simulink model "Hardware_Diagnostics_Test"  (R2025b)
settings: Solver=FixedStepDiscrete  StartTime=0.0  StopTime=inf  FixedStep=50e-6  RelTol=1e-3  EnableMultiTasking=on
undefined symbols (not defined in the file or in its folder): bit, Down, GPTRIP1SEL, GPTRIP2SEL, TZ1, TZ2, Up
libraries: c2802xlib x5, c280xlib x3, c2806xlib x2

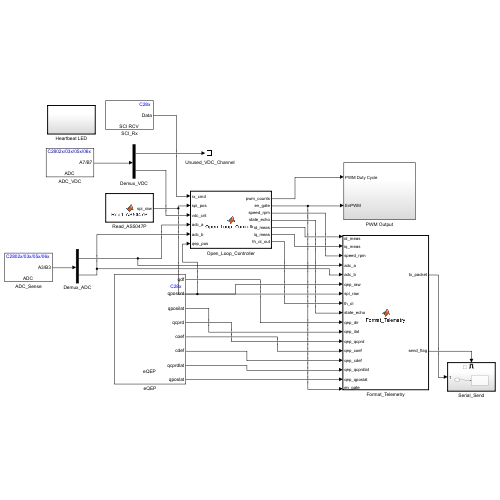
[thumbnail: Simulink's stored preview of the top-level diagram]
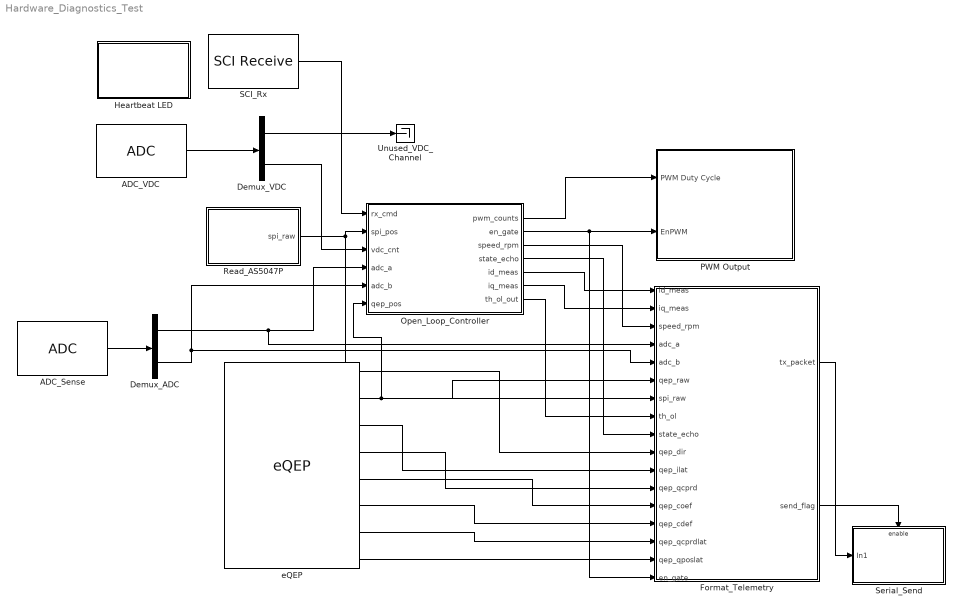
== system Hardware_Diagnostics_Test ==
  ADC_Sense : c2802xlib/ADC  blkParamProc=C2000  ADCModule=1  samplingMode=Simultaneous sample mode  ADCResolution=12-bit (Single-ended input)  ADC29xResolution=12-bit  ADCMode=Single-ended input  useSOC1=SOC0  useSOC2=SOC0_SOC1  SOCAcquisitionWindow=7  SOCTriggerSource=ePWM4_ADCSOCA  SOCInterruptTrigger=No ADCINT  Ts=-1  dType=uint16  postInterrupt=on  interruptSel=ADCINT1  ADCINTContinuous=on  endma=off  chdma=1  conv1=ADCINA0  conv2=ADCINA3 and ADCINB3  conv1_Type4=ADCIN0  conv2_Type4=ADCIN0 and ADCIN1
  ADC_VDC : c2802xlib/ADC  blkParamProc=C2000  ADCModule=1  samplingMode=Simultaneous sample mode  ADCResolution=12-bit (Single-ended input)  ADC29xResolution=12-bit  ADCMode=Single-ended input  useSOC1=SOC2  useSOC2=SOC2_SOC3  SOCAcquisitionWindow=7  SOCTriggerSource=Software  SOCInterruptTrigger=No ADCINT  Ts=-1  dType=uint16  postInterrupt=off  interruptSel=ADCINT1  ADCINTContinuous=on  endma=off  chdma=1  conv1=ADCINB7  conv2=ADCINA7 and ADCINB7  conv1_Type4=ADCIN0  conv2_Type4=ADCIN0 and ADCIN1
  Demux_ADC : Demux  Outputs=2
  Demux_VDC : Demux  Outputs=2
  Format_Telemetry : MATLAB Function  TreatAsAtomicUnit=on
  Heartbeat LED : Subsystem  TreatAsAtomicUnit=on
  Open_Loop_Controller : MATLAB Function  TreatAsAtomicUnit=on
  PWM Output : Subsystem
  Read_AS5047P : MATLAB Function  TreatAsAtomicUnit=on
  SCI_Rx : c280xlib/SCI Receive  Priority=2  sciModule=A  dataHead=''  headerCheckMaxCount=16  dataTail=''  dataType=uint8  dataLenOptions=Length via dialog  dataDim=1  maxDataLength=1  initValue=0  errOption=Output the last received value  errValue=0  sampleTime=-1  blockingMode=off  timeOut=inf  outputStatus=off
  Serial_Send : Subsystem
  Unused_VDC_Channel : Terminator
  eQEP : c280xlib/eQEP  useModule=eQEP1  pcInputmode=Quadrature-count  externalClockrate=2x resolution: Count the rising/falling edge  swapPolarityselection=Counterclockwise  qdfOutputport=on  qapPolarityselection=off  qbpPolarityselection=off  qipPolarityselection=off  qspPolarityselection=off  igatePolarityselection=off  sampleTime=-1  pcOutputport=on  pcMaximumvalue=4095  indexInitializationcheck=off  indexInitializationevent=Falling edge  strobeInitializationcheck=off  strobeInitializationevent=Rising edge  softwareInitializationcheck=off  softwareInitializationsource=Set to init value at start up  softwareInitializationmode=on  pcInitialvalue=0  pcResetmode=Reset on the maximum position  ieloutputport=on  indexEventlatch=Rising edge  seloutputport=off  strobeEventlatch=Rising edge  pcefOutputport=on  enableEqepcapture=on  qctmrOutputport=off  qcprdOutputport=on  captureTimerprescaler=128  upEventprescaler=128  overflowErrorflag=on  directionErrorflag=on  captureTimerposition=On position counter read  unitTimerperiod=100000000  captureTimerlatch=off  capturePeriodlatch=on  positionCounterlatch=on  soenPolarityselection=off  spselPolarityselection=Index pin is used for sync output  compareValuesource=Specify via dialog  shadowMode=Load on QPOSCNT=0  compareValue=4294967295  syncOutputwidth=1  polaritySyncoutput=Active high  watchdogEnable=on  watchdogTimer=65535  outport1Datatype=auto  outport2Datatype=auto  outport3Datatype=auto  outport4Datatype=auto  outport5Datatype=auto  outport6Datatype=auto  outport7Datatype=auto  outport8Datatype=auto  outport9Datatype=auto  outport10Datatype=auto  outport11Datatype=auto  outport12Datatype=auto  eqepinterrupt_pce=on  eqepinterrupt_qpe=on  eqepinterrupt_qdc=on  eqepinterrupt_wto=on  eqepinterrupt_pcu=off  eqepinterrupt_pco=off  eqepinterrupt_pcr=off  eqepinterrupt_pcm=off  eqepinterrupt_sel=off  eqepinterrupt_iel=on  eqepinterrupt_uto=on  pheOutputport=on  watchdogOutputport=on  outport13Datatype=auto  outport14Datatype=auto
  wires:
  ADC_VDC/1 -> Demux_VDC/1
  Demux_VDC/2 -> Open_Loop_Controller/3(vdc_cnt)
  SCI_Rx/1 -> Open_Loop_Controller/1(rx_cmd)
  Open_Loop_Controller/5(id_meas) -> Format_Telemetry/1(id_meas)
  Demux_VDC/1 -> Unused_VDC_Channel/1
  Read_AS5047P/1(spi_raw) -> Format_Telemetry/7(spi_raw), Open_Loop_Controller/2(spi_pos)
  Open_Loop_Controller/1(pwm_counts) -> PWM Output/1(PWM Duty Cycle)
  Open_Loop_Controller/2(en_gate) -> Format_Telemetry/17(en_gate), PWM Output/2(EnPWM)
  Open_Loop_Controller/7(th_ol_out) -> Format_Telemetry/8(th_ol)
  Open_Loop_Controller/3(speed_rpm) -> Format_Telemetry/3(speed_rpm)
  Open_Loop_Controller/4(state_echo) -> Format_Telemetry/9(state_echo)
  Open_Loop_Controller/6(iq_meas) -> Format_Telemetry/2(iq_meas)
  Format_Telemetry/1(tx_packet) -> Serial_Send/1(In1)
  Format_Telemetry/2(send_flag) -> Serial_Send/Enable
  eQEP/8 -> Format_Telemetry/16(qep_qposlat)
  eQEP/6 -> Format_Telemetry/14(qep_cdef)
  eQEP/3 -> Format_Telemetry/11(qep_ilat)
  eQEP/1 -> Format_Telemetry/10(qep_dir)
  eQEP/2 -> Format_Telemetry/6(qep_raw), Open_Loop_Controller/6(qep_pos)
  eQEP/4 -> Format_Telemetry/12(qep_qcprd)
  eQEP/7 -> Format_Telemetry/15(qep_qcprdlat)
  Demux_ADC/1 -> Format_Telemetry/4(adc_a), Open_Loop_Controller/4(adc_a)
  Demux_ADC/2 -> Format_Telemetry/5(adc_b), Open_Loop_Controller/5(adc_b)
  eQEP/5 -> Format_Telemetry/13(qep_coef)
  ADC_Sense/1 -> Demux_ADC/1

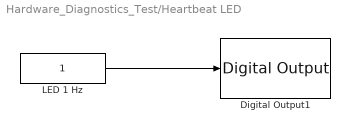
== system Hardware_Diagnostics_Test/Heartbeat LED ==
  Digital Output1 : c2806xlib/Digital Output  GPIO_Number=GPIO32~GPIO39  GPIO_Bit0=off  GPIO_BIT0_Toggle=off  GPIO_Bit1=off  GPIO_BIT1_Toggle=off  GPIO_Bit2=on  GPIO_BIT2_Toggle=on  GPIO_Bit3=off  GPIO_BIT3_Toggle=off  GPIO_Bit4=off  GPIO_BIT4_Toggle=off  GPIO_Bit5=off  GPIO_BIT5_Toggle=off  GPIO_Bit6=off  GPIO_BIT6_Toggle=off  GPIO_Bit7=off  GPIO_BIT7_Toggle=off
  LED 1 Hz : Constant  OutDataTypeStr=uint16  SampleTime=0.5
  wires:
  LED 1 Hz/1 -> Digital Output1/1

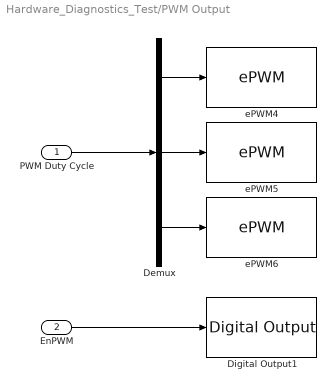
== system Hardware_Diagnostics_Test/PWM Output ==
  PWM Duty Cycle : Inport
  EnPWM : Inport  Port=2
  Demux : Demux  Outputs=3
  Digital Output1 : c2806xlib/Digital Output  GPIO_Number=GPIO50~GPIO55  GPIO_Bit0=off  GPIO_BIT0_Toggle=off  GPIO_Bit1=off  GPIO_BIT1_Toggle=off  GPIO_Bit2=on  GPIO_BIT2_Toggle=off  GPIO_Bit3=off  GPIO_BIT3_Toggle=off  GPIO_Bit4=off  GPIO_BIT4_Toggle=off  GPIO_Bit5=off  GPIO_BIT5_Toggle=off  GPIO_Bit6=off  GPIO_BIT6_Toggle=off  GPIO_Bit7=off  GPIO_BIT7_Toggle=off
  ePWM4 : c2802xlib/ePWM  PwmType=C2000  useModule=ePWM4  ePWMxLINKTBPRD=Not Linked  periodUnits=Clock cycles  timerSource=Specify via dialog  timerPeriod_clk=2250  timerPeriod_sec=64000  tbshadow=Counter equals to zero  countingMode=Up-Down  phaseActiveEnable=Disable  phaseDirection=Count down after sync  phaseActive=0  synchronizationEnable=off  dcaevt1Sync=off  dcbevt1Sync=off  synchronizationOption=Counter equals to zero (CTR=Zero)  dcbevt1SyncOut=off  dcaevt1SyncOut=off  cmpdSyncOut=off  cmpcSyncOut=off  cmpbSyncOut=off  zeroSyncOut=on  swfSyncOut=off  perSynchronizationOption=Counter equals to period (CTR=PRD)  clockPrescale=1  HSclockPrescale=1  enswap=off  ePWMxAStatus=on  ePWMxAactionLogic1=Do nothing  ePWMxAactionLogic2=Do nothing  ePWMxAactionLogic3=Clear  ePWMxAactionLogic4=Set  ePWMxAactionLogic5=Do nothing  ePWMxAactionLogic6=Do nothing  ePWMxACSFenable=off  ePWMxACSFvalue=Forcing disable  ePWMxASFreload=Zero  ePWMxBStatus=off  ePWMxBactionLogic1=Do nothing  ePWMxBactionLogic2=Set  ePWMxBactionLogic3=Do nothing  ePWMxBactionLogic4=Do nothing  ePWMxBactionLogic5=Clear  ePWMxBactionLogic6=Do nothing  ePWMxBCSFenable=off  ePWMxBCSFvalue=Forcing disable  ePWMxBSFreload=Zero  ePWNxBOutWay=off  ePWMxLINKCMPA=Not Linked  CMPAUnits=Clock cycles  CMPASource=Input port  CMPAValue_per=32000  CMPAValue_clk=1125  enCMPAshadow=Counter equals to zero (CTR=Zero)  ePWMxLINKCMPB=Not Linked  CMPBUnits=Clock cycles  CMPBSource=Specify via dialog  CMPBValue_per=50  CMPBValue_clk=1125  enCMPBshadow=Counter equals to zero (CTR=Zero)  ePWMxLINKCMPC=Not Linked  CMPCUnits=Clock cycles  CMPCSource=Specify via dialog  CMPCValue_per=50  CMPCValue_clk=32000  enCMPCshadow=Counter equals to zero (CTR=Zero)  ePWMxLINKCMPD=Not Linked  CMPDUnits=Clock cycles  CMPDSource=Specify via dialog  CMPDValue_per=50  CMPDValue_clk=32000  enCMPDshadow=Counter equals to zero (CTR=Zero)  enableDBePWMxA=on  enableDBePWMxB=on  enhalfcycle=off  DBpolarity=Active high complementary (AHC)  DBedgeDelay=Positive  DBSource_ePWMxA=ePWMxA  DBSource_ePWMxB=ePWMxA  DBPeriodUnits=Clock cycles  DBperiodSource=Specify via dialog  REDperiod=5  FEDperiod=5  REDperiod_sec=0  FEDperiod_sec=0  LoadModeDBRED=Immediate without using shadow  LoadModeDBFED=Immediate without using shadow  adcstartModuleA=on  adcrequestEventA=First event  adcstartEventA=Counter equals to period (CTR=PRD)  adcstartEventA_type2=Digital Compare Module A Event 1 start of conversion (DCAEVT1.soc)  adcstartModuleB=off  adcrequestEventB=First event  adcstartEventB=Counter equals to zero (CTR=Zero)  adcstartEventB_type2=Counter equals to zero (CTR=Zero)  intEn=off  intPrd=First event  intSel=Counter equals to zero (CTR=Zero)  intSel_type2=Counter equals to zero (CTR=Zero)  hrpe=off  enHRPWM=off  HRPWM_LoadMode=Counter equals to period (CTR=PRD)  HRPWM_CTLMode=Duty or Period control mode  HRPWM_EDGMode=Both edge  hrpeb=off  enHRPWMB=off  HRPWM_LoadModeB=Counter equals to zero (CTR=ZERO)  HRPWM_CTLModeB=Duty or Period control mode  HRPWM_EDGModeB=Both edge  enHRDBRED=off  enHRDBFED=off  enSFO=on  enautoconv=on  chopperEnable=off  chopperFrequency=1  chopperFirstwidth=1  chopperDuty=12.5%  tripZonesource=Specify via dialog  tzselOSHT1=off  tzselOSHT2=off  tzselOSHT3=off  tzselOSHT4=off  tzselOSHT5=off  tzselOSHT6=off  tzselOSHDCAEV1=off  tzselOSHDCBEV1=off  tzselCBC1=off  tzselCBC2=off  tzselCBC3=off  tzselCBC4=off  tzselCBC5=off  tzselCBC6=off  tzselCBCDCAEV2=off  tzselCBCDCBEV2=off  enTzOstIntr=off  enTzCbcIntr=off  enTzDCAEVT1Intr=off  enTzDCAEVT2Intr=off  enTzDCBEVT1Intr=off  enTzDCBEVT2Intr=off  tzclrCBCLatch=Counter equals to zero (CTR=Zero)  ePWMxAforced=No action  ePWMxBforced=No action  DCAEVT1forced=No action  DCBEVT1forced=No action  DCAEVT2forced=No action  DCBEVT2forced=No action  dcah=Trip Zone 1 input (TZ1)  dcal=Trip Zone 2 input (TZ2)  dcbh=Trip Zone 1 input (TZ1)  dcbl=Trip Zone 2 input (TZ2)  dcah_type2=GPTRIP1SEL/(TZ1)  dcal_type2=GPTRIP2SEL/(TZ2)  dcbh_type2=GPTRIP1SEL/(TZ1)  dcbl_type2=GPTRIP2SEL/(TZ2)  gendcaevt1=Event disabled  gendcaevt2=Event disabled  gendcbevt1=Event disabled  gendcbevt2=Event disabled  dcaevt1src=DCAEVT1 with sync  dcaevt2src=DCAEVT2 with sync  dcbevt1src=DCBEVT1 with sync  dcbevt2src=DCBEVT2 with sync  pulsesel=Counter equals to zero (CTR=Zero)  blankinv=off  blankoffset=0  blankwidth=0  evsrcsel=Filtered version of DCAEVT1 (DCAEVT1FILT)  encape=off
  ePWM5 : c2802xlib/ePWM  PwmType=C2000  useModule=ePWM5  ePWMxLINKTBPRD=Not Linked  periodUnits=Clock cycles  timerSource=Specify via dialog  timerPeriod_clk=2250  timerPeriod_sec=64000  tbshadow=Counter equals to zero  countingMode=Up-Down  phaseActiveEnable=Set counter to phase value specified via dialog  phaseDirection=Count up after sync  phaseActive=0  synchronizationEnable=off  dcaevt1Sync=off  dcbevt1Sync=off  synchronizationOption=Pass through (EPWMxSYNCI or SWFSYNC)  dcbevt1SyncOut=off  dcaevt1SyncOut=off  cmpdSyncOut=off  cmpcSyncOut=off  cmpbSyncOut=off  zeroSyncOut=off  swfSyncOut=on  perSynchronizationOption=Counter equals to period (CTR=PRD)  clockPrescale=1  HSclockPrescale=1  enswap=off  ePWMxAStatus=on  ePWMxAactionLogic1=Do nothing  ePWMxAactionLogic2=Do nothing  ePWMxAactionLogic3=Clear  ePWMxAactionLogic4=Set  ePWMxAactionLogic5=Do nothing  ePWMxAactionLogic6=Do nothing  ePWMxACSFenable=off  ePWMxACSFvalue=Forcing disable  ePWMxASFreload=Zero  ePWMxBStatus=off  ePWMxBactionLogic1=Do nothing  ePWMxBactionLogic2=Set  ePWMxBactionLogic3=Do nothing  ePWMxBactionLogic4=Do nothing  ePWMxBactionLogic5=Clear  ePWMxBactionLogic6=Do nothing  ePWMxBCSFenable=off  ePWMxBCSFvalue=Forcing disable  ePWMxBSFreload=Zero  ePWNxBOutWay=off  ePWMxLINKCMPA=Not Linked  CMPAUnits=Clock cycles  CMPASource=Input port  CMPAValue_per=32000  CMPAValue_clk=1125  enCMPAshadow=Counter equals to zero (CTR=Zero)  ePWMxLINKCMPB=Not Linked  CMPBUnits=Clock cycles  CMPBSource=Specify via dialog  CMPBValue_per=50  CMPBValue_clk=1125  enCMPBshadow=Counter equals to zero (CTR=Zero)  ePWMxLINKCMPC=Not Linked  CMPCUnits=Clock cycles  CMPCSource=Specify via dialog  CMPCValue_per=50  CMPCValue_clk=32000  enCMPCshadow=Counter equals to zero (CTR=Zero)  ePWMxLINKCMPD=Not Linked  CMPDUnits=Clock cycles  CMPDSource=Specify via dialog  CMPDValue_per=50  CMPDValue_clk=32000  enCMPDshadow=Counter equals to zero (CTR=Zero)  enableDBePWMxA=on  enableDBePWMxB=on  enhalfcycle=off  DBpolarity=Active high complementary (AHC)  DBedgeDelay=Positive  DBSource_ePWMxA=ePWMxA  DBSource_ePWMxB=ePWMxA  DBPeriodUnits=Clock cycles  DBperiodSource=Specify via dialog  REDperiod=5  FEDperiod=5  REDperiod_sec=0  FEDperiod_sec=0  LoadModeDBRED=Immediate without using shadow  LoadModeDBFED=Immediate without using shadow  adcstartModuleA=off  adcrequestEventA=First event  adcstartEventA=Digital Compare Module A Event 1 start of conversion (DCAEVT1.soc)  adcstartEventA_type2=Digital Compare Module A Event 1 start of conversion (DCAEVT1.soc)  adcstartModuleB=off  adcrequestEventB=First event  adcstartEventB=Counter equals to zero (CTR=Zero)  adcstartEventB_type2=Counter equals to zero (CTR=Zero)  intEn=off  intPrd=First event  intSel=Counter equals to zero (CTR=Zero)  intSel_type2=Counter equals to zero (CTR=Zero)  hrpe=off  enHRPWM=off  HRPWM_LoadMode=Counter equals to period (CTR=PRD)  HRPWM_CTLMode=Duty or Period control mode  HRPWM_EDGMode=Both edge  hrpeb=off  enHRPWMB=off  HRPWM_LoadModeB=Counter equals to zero (CTR=ZERO)  HRPWM_CTLModeB=Duty or Period control mode  HRPWM_EDGModeB=Both edge  enHRDBRED=off  enHRDBFED=off  enSFO=on  enautoconv=on  chopperEnable=off  chopperFrequency=1  chopperFirstwidth=1  chopperDuty=12.5%  tripZonesource=Specify via dialog  tzselOSHT1=off  tzselOSHT2=off  tzselOSHT3=off  tzselOSHT4=off  tzselOSHT5=off  tzselOSHT6=off  tzselOSHDCAEV1=off  tzselOSHDCBEV1=off  tzselCBC1=off  tzselCBC2=off  tzselCBC3=off  tzselCBC4=off  tzselCBC5=off  tzselCBC6=off  tzselCBCDCAEV2=off  tzselCBCDCBEV2=off  enTzOstIntr=off  enTzCbcIntr=off  enTzDCAEVT1Intr=off  enTzDCAEVT2Intr=off  enTzDCBEVT1Intr=off  enTzDCBEVT2Intr=off  tzclrCBCLatch=Counter equals to zero (CTR=Zero)  ePWMxAforced=No action  ePWMxBforced=No action  DCAEVT1forced=No action  DCBEVT1forced=No action  DCAEVT2forced=No action  DCBEVT2forced=No action  dcah=Trip Zone 1 input (TZ1)  dcal=Trip Zone 2 input (TZ2)  dcbh=Trip Zone 1 input (TZ1)  dcbl=Trip Zone 2 input (TZ2)  dcah_type2=GPTRIP1SEL/(TZ1)  dcal_type2=GPTRIP2SEL/(TZ2)  dcbh_type2=GPTRIP1SEL/(TZ1)  dcbl_type2=GPTRIP2SEL/(TZ2)  gendcaevt1=Event disabled  gendcaevt2=Event disabled  gendcbevt1=Event disabled  gendcbevt2=Event disabled  dcaevt1src=DCAEVT1 with sync  dcaevt2src=DCAEVT2 with sync  dcbevt1src=DCBEVT1 with sync  dcbevt2src=DCBEVT2 with sync  pulsesel=Counter equals to zero (CTR=Zero)  blankinv=off  blankoffset=0  blankwidth=0  evsrcsel=Filtered version of DCAEVT1 (DCAEVT1FILT)  encape=off
  ePWM6 : c2802xlib/ePWM  PwmType=C2000  useModule=ePWM6  ePWMxLINKTBPRD=Not Linked  periodUnits=Clock cycles  timerSource=Specify via dialog  timerPeriod_clk=2250  timerPeriod_sec=64000  tbshadow=Counter equals to zero  countingMode=Up-Down  phaseActiveEnable=Set counter to phase value specified via dialog  phaseDirection=Count up after sync  phaseActive=0  synchronizationEnable=off  dcaevt1Sync=off  dcbevt1Sync=off  synchronizationOption=Disable  dcbevt1SyncOut=off  dcaevt1SyncOut=off  cmpdSyncOut=off  cmpcSyncOut=off  cmpbSyncOut=off  zeroSyncOut=off  swfSyncOut=off  perSynchronizationOption=Counter equals to period (CTR=PRD)  clockPrescale=1  HSclockPrescale=1  enswap=off  ePWMxAStatus=on  ePWMxAactionLogic1=Do nothing  ePWMxAactionLogic2=Do nothing  ePWMxAactionLogic3=Clear  ePWMxAactionLogic4=Set  ePWMxAactionLogic5=Do nothing  ePWMxAactionLogic6=Do nothing  ePWMxACSFenable=off  ePWMxACSFvalue=Forcing disable  ePWMxASFreload=Zero  ePWMxBStatus=off  ePWMxBactionLogic1=Do nothing  ePWMxBactionLogic2=Set  ePWMxBactionLogic3=Do nothing  ePWMxBactionLogic4=Do nothing  ePWMxBactionLogic5=Clear  ePWMxBactionLogic6=Do nothing  ePWMxBCSFenable=off  ePWMxBCSFvalue=Forcing disable  ePWMxBSFreload=Zero  ePWNxBOutWay=off  ePWMxLINKCMPA=Not Linked  CMPAUnits=Clock cycles  CMPASource=Input port  CMPAValue_per=32000  CMPAValue_clk=1125  enCMPAshadow=Counter equals to zero (CTR=Zero)  ePWMxLINKCMPB=Not Linked  CMPBUnits=Clock cycles  CMPBSource=Specify via dialog  CMPBValue_per=50  CMPBValue_clk=1125  enCMPBshadow=Counter equals to zero (CTR=Zero)  ePWMxLINKCMPC=Not Linked  CMPCUnits=Clock cycles  CMPCSource=Specify via dialog  CMPCValue_per=50  CMPCValue_clk=32000  enCMPCshadow=Counter equals to zero (CTR=Zero)  ePWMxLINKCMPD=Not Linked  CMPDUnits=Clock cycles  CMPDSource=Specify via dialog  CMPDValue_per=50  CMPDValue_clk=32000  enCMPDshadow=Counter equals to zero (CTR=Zero)  enableDBePWMxA=on  enableDBePWMxB=on  enhalfcycle=off  DBpolarity=Active high complementary (AHC)  DBedgeDelay=Positive  DBSource_ePWMxA=ePWMxA  DBSource_ePWMxB=ePWMxA  DBPeriodUnits=Clock cycles  DBperiodSource=Specify via dialog  REDperiod=5  FEDperiod=5  REDperiod_sec=0  FEDperiod_sec=0  LoadModeDBRED=Immediate without using shadow  LoadModeDBFED=Immediate without using shadow  adcstartModuleA=off  adcrequestEventA=First event  adcstartEventA=Digital Compare Module A Event 1 start of conversion (DCAEVT1.soc)  adcstartEventA_type2=Digital Compare Module A Event 1 start of conversion (DCAEVT1.soc)  adcstartModuleB=off  adcrequestEventB=First event  adcstartEventB=Counter equals to zero (CTR=Zero)  adcstartEventB_type2=Counter equals to zero (CTR=Zero)  intEn=off  intPrd=First event  intSel=Counter equals to zero (CTR=Zero)  intSel_type2=Counter equals to zero (CTR=Zero)  hrpe=off  enHRPWM=off  HRPWM_LoadMode=Counter equals to period (CTR=PRD)  HRPWM_CTLMode=Duty or Period control mode  HRPWM_EDGMode=Both edge  hrpeb=off  enHRPWMB=off  HRPWM_LoadModeB=Counter equals to zero (CTR=ZERO)  HRPWM_CTLModeB=Duty or Period control mode  HRPWM_EDGModeB=Both edge  enHRDBRED=off  enHRDBFED=off  enSFO=on  enautoconv=on  chopperEnable=off  chopperFrequency=1  chopperFirstwidth=1  chopperDuty=12.5%  tripZonesource=Specify via dialog  tzselOSHT1=off  tzselOSHT2=off  tzselOSHT3=off  tzselOSHT4=off  tzselOSHT5=off  tzselOSHT6=off  tzselOSHDCAEV1=off  tzselOSHDCBEV1=off  tzselCBC1=off  tzselCBC2=off  tzselCBC3=off  tzselCBC4=off  tzselCBC5=off  tzselCBC6=off  tzselCBCDCAEV2=off  tzselCBCDCBEV2=off  enTzOstIntr=off  enTzCbcIntr=off  enTzDCAEVT1Intr=off  enTzDCAEVT2Intr=off  enTzDCBEVT1Intr=off  enTzDCBEVT2Intr=off  tzclrCBCLatch=Counter equals to zero (CTR=Zero)  ePWMxAforced=No action  ePWMxBforced=No action  DCAEVT1forced=No action  DCBEVT1forced=No action  DCAEVT2forced=No action  DCBEVT2forced=No action  dcah=Trip Zone 1 input (TZ1)  dcal=Trip Zone 2 input (TZ2)  dcbh=Trip Zone 1 input (TZ1)  dcbl=Trip Zone 2 input (TZ2)  dcah_type2=GPTRIP1SEL/(TZ1)  dcal_type2=GPTRIP2SEL/(TZ2)  dcbh_type2=GPTRIP1SEL/(TZ1)  dcbl_type2=GPTRIP2SEL/(TZ2)  gendcaevt1=Event disabled  gendcaevt2=Event disabled  gendcbevt1=Event disabled  gendcbevt2=Event disabled  dcaevt1src=DCAEVT1 with sync  dcaevt2src=DCAEVT2 with sync  dcbevt1src=DCBEVT1 with sync  dcbevt2src=DCBEVT2 with sync  pulsesel=Counter equals to zero (CTR=Zero)  blankinv=off  blankoffset=0  blankwidth=0  evsrcsel=Filtered version of DCAEVT1 (DCAEVT1FILT)  encape=off
  wires:
  Demux/1 -> ePWM4/1
  Demux/2 -> ePWM5/1
  PWM Duty Cycle/1 -> Demux/1
  Demux/3 -> ePWM6/1
  EnPWM/1 -> Digital Output1/1

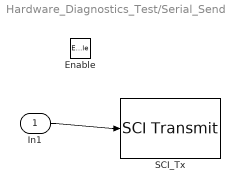
== system Hardware_Diagnostics_Test/Serial_Send ==
  In1 : Inport
  Enable : EnablePort
  SCI_Tx : c280xlib/SCI Transmit  sciModule=A  dataHead='S'  dataTail='E'  frameSize=1  blockingMode=on  outputStatus=off
  wires:
  In1/1 -> SCI_Tx/1

== matlab function Hardware_Diagnostics_Test/Read_AS5047P ==
function spi_raw = Read_AS5047P()
%#codegen
% SPI-A AS5047P read on GPIO16/17/18 with GPIO19 chip select.
% Force the EPC91200 PWM trip before the first controller update.
persistent init_done
spi_raw = uint16(0);
if coder.target('Rtw')
    coder.cinclude('as5047p_spi.h');
    coder.cinclude('pwm_gate_control.h');
    coder.updateBuildInfo('addSourceFiles', 'as5047p_spi.c');
    coder.updateBuildInfo('addSourceFiles', 'pwm_gate_control.c');
    coder.updateBuildInfo('addIncludePaths', 'C:\\96v_gan_humanoid_drive\\phase1\\simulation\\MyFOC code');
    if isempty(init_done)
        coder.ceval('pwm_gate_control', uint16(0));
        coder.ceval('as5047p_spi_init');
        init_done = true;
    end
    coder.ceval('as5047p_spi_read', coder.ref(spi_raw));
end
end

== matlab function Hardware_Diagnostics_Test/Format_Telemetry ==
function [tx_packet, send_flag] = Format_Telemetry(id_meas, iq_meas, speed_rpm, adc_a, adc_b, qep_raw, spi_raw, th_ol, state_echo, qep_dir, qep_ilat, qep_qcprd, qep_coef, qep_cdef, qep_qcprdlat, qep_qposlat, en_gate)
%#codegen
persistent dec_cnt
if isempty(dec_cnt), dec_cnt=uint16(0); end
dec_cnt=dec_cnt+uint16(1);
if dec_cnt>=uint16(20), dec_cnt=uint16(0); send_flag=true; else, send_flag=false; end

tx_packet=zeros(33,1,'uint8');
id_u16=typecast(int16(round(id_meas*single(100.0))),'uint16');
iq_u16=typecast(int16(round(iq_meas*single(100.0))),'uint16');
spd_u16=typecast(int16(round(speed_rpm)),'uint16');
aa=uint16(adc_a); ab=uint16(adc_b); spi_val=uint16(spi_raw); qep_val=uint16(qep_raw); ilat_val=uint16(qep_ilat);
th_norm=th_ol*single(10430.37835); if th_norm<single(0.0), th_norm=single(0.0); end; if th_norm>single(65535.0), th_norm=single(65535.0); end; th_u16=uint16(th_norm);
qcprd_val=uint16(qep_qcprd); coef_val=uint16(qep_coef); cdef_val=uint16(qep_cdef); qcprdlat_val=uint16(qep_qcprdlat); qposlat_val=uint16(qep_qposlat);

tx_packet(1)=uint8(83); tx_packet(2)=uint8(170); tx_packet(3)=uint8(85);
tx_packet(4)=uint8(bitshift(id_u16,-8)); tx_packet(5)=uint8(bitand(id_u16,255)); tx_packet(6)=uint8(bitshift(iq_u16,-8)); tx_packet(7)=uint8(bitand(iq_u16,255)); tx_packet(8)=uint8(bitshift(spd_u16,-8)); tx_packet(9)=uint8(bitand(spd_u16,255));
tx_packet(10)=uint8(bitshift(aa,-8)); tx_packet(11)=uint8(bitand(aa,255)); tx_packet(12)=uint8(bitshift(ab,-8)); tx_packet(13)=uint8(bitand(ab,255)); tx_packet(14)=uint8(bitshift(spi_val,-8)); tx_packet(15)=uint8(bitand(spi_val,255)); tx_packet(16)=uint8(bitshift(qep_val,-8)); tx_packet(17)=uint8(bitand(qep_val,255));
tx_packet(18)=uint8(bitshift(ilat_val,-8)); tx_packet(19)=uint8(bitand(ilat_val,255)); tx_packet(20)=uint8(qep_dir~=0); tx_packet(21)=uint8(qep_coef~=0); tx_packet(22)=uint8(qep_cdef~=0);
tx_packet(23)=uint8(bitshift(qcprd_val,-8)); tx_packet(24)=uint8(bitand(qcprd_val,255)); tx_packet(25)=uint8(bitshift(qcprdlat_val,-8)); tx_packet(26)=uint8(bitand(qcprdlat_val,255)); tx_packet(27)=uint8(bitshift(qposlat_val,-8)); tx_packet(28)=uint8(bitand(qposlat_val,255));
tx_packet(29)=uint8(bitshift(th_u16,-8)); tx_packet(30)=uint8(bitand(th_u16,255)); tx_packet(31)=uint8(state_echo); tx_packet(32)=uint8(en_gate); tx_packet(33)=uint8(69);
end

== matlab function Hardware_Diagnostics_Test/Open_Loop_Controller ==
function [pwm_counts, en_gate, speed_rpm, state_echo, id_meas, iq_meas, th_ol_out] = Open_Loop_Controller(rx_cmd, spi_pos, vdc_cnt, adc_a, adc_b, qep_pos)
%#codegen
% BOARD-SIDE COMMISSIONING CONTROLLER
%
% Commands:
%   0/S/s : stop and latch the ePWM software trip
%   A/a/4 : apply a small static alignment vector and capture both encoders
%   P/p/5 : open-loop electrical rotation in the board-positive direction
%   N/n/7 : open-loop electrical rotation in the board-negative direction
%   C/c   : clear the captured QEP electrical offset and stop
%
% SPI is sampled during alignment as an independent absolute reference.
% QEP is the runtime mechanical angle/speed source after calibration.
% The dashboard does not alter any of these signs.

pwm_counts = single([1125.0;1125.0;1125.0]);
en_gate = false;
speed_rpm = single(0.0);
state_echo = uint8(0);
id_meas = single(0.0);
iq_meas = single(0.0);
th_ol_out = single(0.0);

persistent state align_timer sample_count sum_spi_sin sum_spi_cos ...
    sum_qep_sin sum_qep_cos qep_elec_offset cal_valid spd_timer ...
    last_qep filt_speed qep_speed_initialized theta_ol last_cmd

if isempty(state)
    state = uint8(0);
    align_timer = uint32(0);
    sample_count = uint32(0);
    sum_spi_sin = single(0.0);
    sum_spi_cos = single(0.0);
    sum_qep_sin = single(0.0);
    sum_qep_cos = single(0.0);
    qep_elec_offset = single(0.0);
    cal_valid = false;
    spd_timer = uint16(0);
    last_qep = uint16(0);
    filt_speed = single(0.0);
    qep_speed_initialized = false;
    theta_ol = single(0.0);
    last_cmd = uint8(0);
end

TWO_PI = single(6.283185307);
TWO_PI_OVER_3 = single(2.094395102);
POLE_PAIRS = single(21.0);
SPI_COUNTS_PER_REV = single(16384.0);
QEP_COUNTS_PER_REV = int32(4096);
QEP_HALF_REV = int32(2048);
QEP_ANGLE_SCALE = TWO_PI / single(4096.0);
QEP_RPM_SCALE = single(14.6484375);       % 4096 counts/rev, 1 ms update
TS_FAST = single(0.00005);                 % 20 kHz controller step
PWM_PERIOD = single(2250.0);

ALIGN_HOLD_TICKS = uint32(30000);          % 1.5 s
ALIGN_SETTLE_TICKS = uint32(20000);        % collect after first 1.0 s
ALIGN_MIN_SAMPLES = uint32(500);
ALIGN_MODULATION = single(0.01);            % intentionally conservative
OPEN_LOOP_MODULATION = single(0.02);        % first powered test only
OPEN_LOOP_MECH_RPM = single(2.0);            % deliberately slow bench test
OPEN_LOOP_ELEC_SPEED = OPEN_LOOP_MECH_RPM * POLE_PAIRS * TWO_PI / single(60.0);
ALIGN_CURRENT_LIMIT = single(1.0);          % board ADC units must be verified
MIN_VDC = single(30.0);

% Convert board ADC channels to the existing diagnostic current estimate.
vdc_volts = single(vdc_cnt) * single(3.3 * 46.4545 / 4095.0);
offset_a = single(2041.0);
offset_b = single(2059.0);
I_SCALE = single(-0.02014652);
ia = (single(adc_a) - offset_a) * I_SCALE;
ib = (single(adc_b) - offset_b) * I_SCALE;
i_alpha = ia;
i_beta = (ia + single(2.0) * ib) * single(0.577350269);
i_mag = sqrt(i_alpha * i_alpha + i_beta * i_beta);

% Raw encoder angles. QEP polarity was configured in the model so the
% hand-spin-positive direction is the board-positive direction.
spi_i32 = mod(int32(spi_pos), int32(16384));
if spi_i32 < int32(0), spi_i32 = spi_i32 + int32(16384); end
theta_spi = single(spi_i32) / SPI_COUNTS_PER_REV * TWO_PI;

qep_i32 = mod(int32(qep_pos), QEP_COUNTS_PER_REV);
if qep_i32 < int32(0), qep_i32 = qep_i32 + QEP_COUNTS_PER_REV; end
theta_qep = single(qep_i32) * QEP_ANGLE_SCALE;

% QEP speed with a first-sample guard so startup cannot create false RPM.
if ~qep_speed_initialized
    last_qep = uint16(qep_i32);
    qep_speed_initialized = true;
end
spd_timer = spd_timer + uint16(1);
if spd_timer >= uint16(20)
    spd_timer = uint16(0);
    delta_qep = qep_i32 - int32(last_qep);
    if delta_qep > QEP_HALF_REV
        delta_qep = delta_qep - QEP_COUNTS_PER_REV;
    elseif delta_qep < -QEP_HALF_REV
        delta_qep = delta_qep + QEP_COUNTS_PER_REV;
    end
    last_qep = uint16(qep_i32);
    filt_speed = single(0.85) * filt_speed + ...
        single(0.15) * single(delta_qep) * QEP_RPM_SCALE;
end
speed_rpm = filt_speed;

% Process command bytes. A zero/no-byte result is ignored so a command
% remains latched until the next explicit command or STOP.
last_state = state;
% Execute each recognized serial command once. This prevents a held SCI byte
% from restarting alignment on every 50 us step.
if rx_cmd ~= last_cmd
    if rx_cmd == uint8(48) || rx_cmd == uint8(83) || rx_cmd == uint8(115)
        state = uint8(0);
        last_cmd = rx_cmd;
    elseif rx_cmd == uint8(65) || rx_cmd == uint8(97) || rx_cmd == uint8(52)
        state = uint8(4);
        last_cmd = rx_cmd;
    elseif rx_cmd == uint8(80) || rx_cmd == uint8(112) || rx_cmd == uint8(53)
        state = uint8(5);
        last_cmd = rx_cmd;
    elseif rx_cmd == uint8(78) || rx_cmd == uint8(110) || rx_cmd == uint8(55)
        state = uint8(7);
        last_cmd = rx_cmd;
    elseif rx_cmd == uint8(67) || rx_cmd == uint8(99)
        state = uint8(0);
        cal_valid = false;
        qep_elec_offset = single(0.0);
        theta_ol = single(0.0);
        last_cmd = rx_cmd;
    end
end

if state ~= last_state
    if state == uint8(4)
        align_timer = uint32(0);
        sample_count = uint32(0);
        sum_spi_sin = single(0.0);
        sum_spi_cos = single(0.0);
        sum_qep_sin = single(0.0);
        sum_qep_cos = single(0.0);
    elseif state == uint8(5) || state == uint8(7)
        % Start at the measured QEP electrical position so a re-run after
        % a hand movement is deterministic.
        theta_qep_e = mod(POLE_PAIRS * theta_qep + qep_elec_offset + TWO_PI, TWO_PI);
        theta_ol = theta_qep_e;
    end
end

% Runtime electrical angle from calibrated QEP. This is intentionally not
% derived from SPI during the open-loop test.
theta_qep_e = mod(POLE_PAIRS * theta_qep + qep_elec_offset + TWO_PI, TWO_PI);
cos_qep_e = cos(theta_qep_e);
sin_qep_e = sin(theta_qep_e);
id_meas = i_alpha * cos_qep_e + i_beta * sin_qep_e;
iq_meas = -i_alpha * sin_qep_e + i_beta * cos_qep_e;

if state == uint8(4)
    state_echo = uint8(4);
    if vdc_volts < MIN_VDC
        state_echo = uint8(13);             % requested alignment, no HV bus
        en_gate = false;
        pwm_counts = single([1125.0;1125.0;1125.0]);
    elseif i_mag > ALIGN_CURRENT_LIMIT
        state = uint8(11);
        state_echo = uint8(11);
        en_gate = false;
        pwm_counts = single([1125.0;1125.0;1125.0]);
    else
        align_timer = align_timer + uint32(1);

        % Static positive phase-A vector: electrical zero for this test.
        da = single(0.5) + ALIGN_MODULATION;
        db = single(0.5) - ALIGN_MODULATION * single(0.5);
        dc = db;
        pwm_counts = [da * PWM_PERIOD; db * PWM_PERIOD; dc * PWM_PERIOD];
        en_gate = true;

        if align_timer >= ALIGN_SETTLE_TICKS
            sum_spi_sin = sum_spi_sin + sin(theta_spi);
            sum_spi_cos = sum_spi_cos + cos(theta_spi);
            sum_qep_sin = sum_qep_sin + sin(theta_qep);
            sum_qep_cos = sum_qep_cos + cos(theta_qep);
            sample_count = sample_count + uint32(1);
        end

        if align_timer >= ALIGN_HOLD_TICKS
            if sample_count >= ALIGN_MIN_SAMPLES && ...
                    abs(sum_qep_sin) + abs(sum_qep_cos) > single(1.0) && ...
                    abs(sum_spi_sin) + abs(sum_spi_cos) > single(1.0)
                qep_mean = atan2(sum_qep_sin, sum_qep_cos);
                if qep_mean < single(0.0), qep_mean = qep_mean + TWO_PI; end
                % At alignment, the commanded phase-A vector is electrical 0.
                qep_elec_offset = mod(-POLE_PAIRS * qep_mean + TWO_PI, TWO_PI);
                cal_valid = true;
                state = uint8(10);
                state_echo = uint8(10);
                en_gate = false;
                pwm_counts = single([1125.0;1125.0;1125.0]);
            else
                state = uint8(12);
                state_echo = uint8(12);
                en_gate = false;
                pwm_counts = single([1125.0;1125.0;1125.0]);
            end
        end
    end
elseif state == uint8(5) || state == uint8(7)
    if ~cal_valid
        state_echo = uint8(8);                % align first
        en_gate = false;
        pwm_counts = single([1125.0;1125.0;1125.0]);
    elseif vdc_volts < MIN_VDC
        state_echo = uint8(13);               % no HV bus
        en_gate = false;
        pwm_counts = single([1125.0;1125.0;1125.0]);
    elseif i_mag > ALIGN_CURRENT_LIMIT
        state = uint8(11);
        state_echo = uint8(11);
        en_gate = false;
        pwm_counts = single([1125.0;1125.0;1125.0]);
    else
        if state == uint8(5)
            theta_ol = theta_ol + OPEN_LOOP_ELEC_SPEED * TS_FAST;
        else
            theta_ol = theta_ol - OPEN_LOOP_ELEC_SPEED * TS_FAST;
        end
        if theta_ol >= TWO_PI
            theta_ol = theta_ol - TWO_PI;
        elseif theta_ol < single(0.0)
            theta_ol = theta_ol + TWO_PI;
        end

        da = single(0.5) + OPEN_LOOP_MODULATION * cos(theta_ol);
        db = single(0.5) + OPEN_LOOP_MODULATION * cos(theta_ol - TWO_PI_OVER_3);
        dc = single(0.5) + OPEN_LOOP_MODULATION * cos(theta_ol + TWO_PI_OVER_3);
        pwm_counts = [da * PWM_PERIOD; db * PWM_PERIOD; dc * PWM_PERIOD];
        en_gate = true;
        state_echo = state;
    end
else
    % Stopped, valid calibration, or latched fault: software ePWM trip is
    % the actual gate-off mechanism. Neutral compare values are retained
    % because CMPA=0 is not a safe disable for complementary PWM.
    en_gate = false;
    pwm_counts = single([1125.0;1125.0;1125.0]);
    if state == uint8(10) || (state == uint8(0) && cal_valid)
        state_echo = uint8(10);
    elseif state == uint8(11)
        state_echo = uint8(11);
    elseif state == uint8(12)
        state_echo = uint8(12);
    else
        state_echo = uint8(0);
    end
end

if state == uint8(10) || (state == uint8(0) && cal_valid)
    th_ol_out = qep_elec_offset;
elseif state == uint8(5) || state == uint8(7)
    th_ol_out = theta_ol;
else
    th_ol_out = theta_spi;
end

% EPC91200 has no usable nEN gate-disable path in this wiring. Force the
% ePWM trip from the controller itself; GPIO52 is only a legacy diagnostic.
if coder.target('Rtw')
    coder.cinclude('pwm_gate_control.h');
    coder.updateBuildInfo('addSourceFiles', 'pwm_gate_control.c');
    coder.updateBuildInfo('addIncludePaths', 'C:\\96v_gan_humanoid_drive\\phase1\\simulation\\MyFOC code');
    gate_cmd = uint16(en_gate);
    coder.ceval('pwm_gate_control', gate_cmd);
end
end
